simulink model "InverterStartupControl"  (R2022b)
settings: Solver=FixedStepAuto  StartTime=0.0  StopTime=inf  FixedStep=0.005  RelTol=1e-3  EnableMultiTasking=on
undefined symbols (not defined in the file or in its folder): canChannel
libraries: canmsglib x6, canlib x3, simulink x1, motor_interface_lib x1, realtime_pacer_lib x1
settings Model: ExtModeTrigDuration=10  Creator=LinF  LastModifiedBy=LinF
settings SolverCC: AutoInsertRateTranBlk=on
settings OptimizationCC: EnhancedBackFolding=on  PassReuseOutputArgsAs=Individual arguments  ZeroExternalMemoryAtStartup=off  ZeroInternalMemoryAtStartup=off  MaxStackSize=64  OptimizeBlockOrder=speed  DifferentSizesBufferReuse=on  OptimizationCustomize=off  EfficientTunableParamExpr=on
settings DebuggingCC: ParameterTunabilityLossMsg=error
settings HardwareCC: ProdBitPerPointer=32  ProdBitPerSizeT=32  ProdBitPerPtrDiffT=32  ProdLargestAtomicInteger=Long  ProdLargestAtomicFloat=Double  ProdWordSize=32  ProdLongLongMode=on  ProdHWDeviceType=ARM Compatible->ARM Cortex  UseEmbeddedCoderFeatures=off
settings SFSimCC: MATLABDynamicMemAlloc=off
settings RTWCC: Description=Embedded Coder  SystemTargetFile=ert.tlc  HardwareBoard=STM32 Nucleo F767ZI  TLCOptions=-aInlineSetEventsForThisBaseRateFcn=TLC_FALSE -aSuppressMultiTaskScheduler=TLC_FALSE -aRateBasedStepFcn=1  TemplateMakefile=ert_default_tmf  Toolchain=GNU Tools for ARM Embedded Processors
settings CodeAppCC: ForceParamTrailComments=on  IgnoreCustomStorageClasses=off  OperatorAnnotations=on  SimulinkDataObjDesc=on  SFDataObjDesc=on  InsertBlockDesc=on
settings ERTTargetCC: SupportNonInlinedSFcns=on  ExtModeTransport=3  ExtModeStaticAlloc=on  ExtModeStaticAllocSize=2000  ExtModeMexFile=ext_xcp  ExtModeIntrfLevel=Level2 - Open

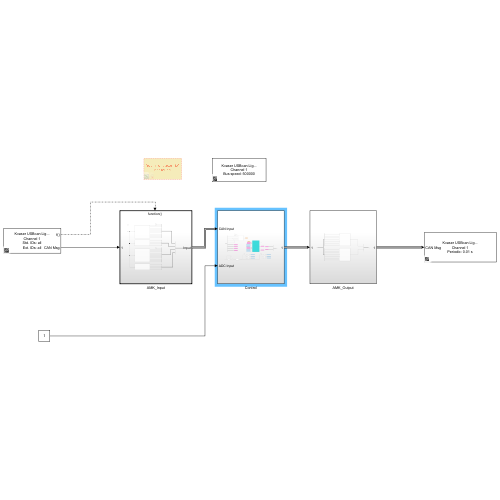
[thumbnail: Simulink's stored preview of the top-level diagram]
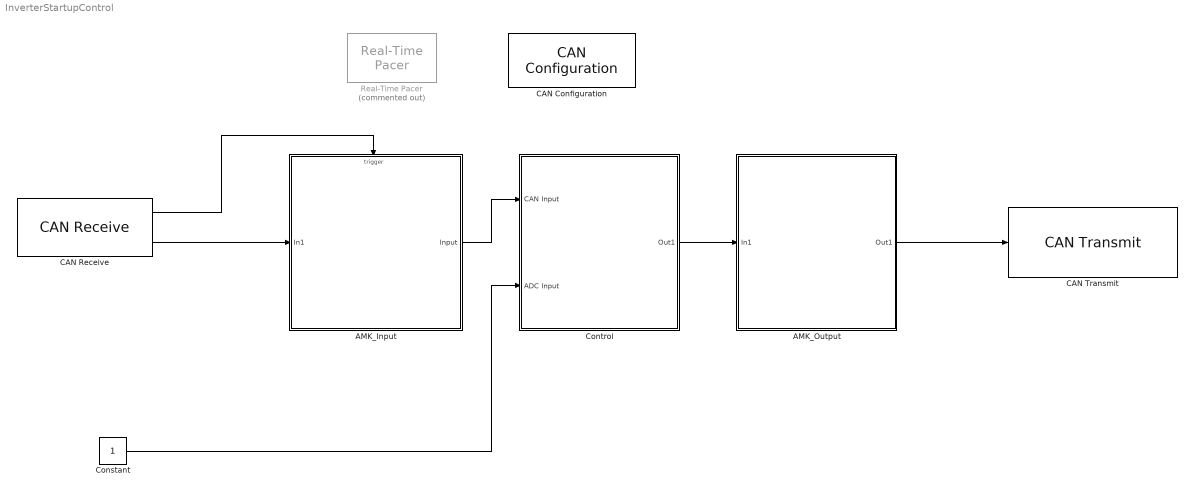
== system InverterStartupControl ==
  AMK_Input : Subsystem  TreatAsAtomicUnit=on
  AMK_Output : Subsystem
  CAN Configuration : canlib/CAN Configuration  BlockHandle=168.0002  Device=Kvaser USBcan Light 1 (Channel 1)  DeviceMenu=Kvaser USBcan Light 1 (Channel 1)  ObjConstructor=canChannel('Kvaser', 'USBcan Light 1', 1)  BusSpeed=500000  EnableBitParameters=off  SJW=4  TSEG1=11  TSEG2=4  NSamples=3  AckMode=Normal
  CAN Receive : canlib/CAN Receive  BlockHandle=169.0002  Device=Kvaser USBcan Light 1 (Channel 1)  DeviceMenu=Kvaser USBcan Light 1 (Channel 1)  ObjConstructor=canChannel('Kvaser', 'USBcan Light 1', 1)  EnableStandardIDsFilter=off  StdIDsCombo=Allow all  StandardIDs=0  EnableExtendedIDsFilter=off  ExtIDsCombo=Allow all  ExtendedIDs=0  SampleTime=0.005  MsgsPerTimestep=all  InternalFilterUpdateStatus=on  BusOutput=off
  CAN Transmit : canlib/CAN Transmit  BlockHandle=172.0002  Device=Kvaser USBcan Light 1 (Channel 1)  DeviceMenu=Kvaser USBcan Light 1 (Channel 1)  ObjConstructor=canChannel('Kvaser', 'USBcan Light 1', 1)  EnableEventTransmit=off  EnablePeriodicTransmit=on  MessagePeriod=0.01
  Constant : Constant
  Control : Subsystem
  Real-Time Pacer : realtime_pacer_lib/Real-Time Pacer  Commented=on  simTimePerRealTime=1
  wires:
  Control/1(Out1) -> AMK_Output/1(In1)
  AMK_Input/1(Input) -> Control/1(CAN Input)
  AMK_Output/1(Out1) -> CAN Transmit/1
  CAN Receive/2 -> AMK_Input/1(In1)
  CAN Receive/1 -> AMK_Input/Trigger
  Constant/1 -> Control/2(ADC Input)

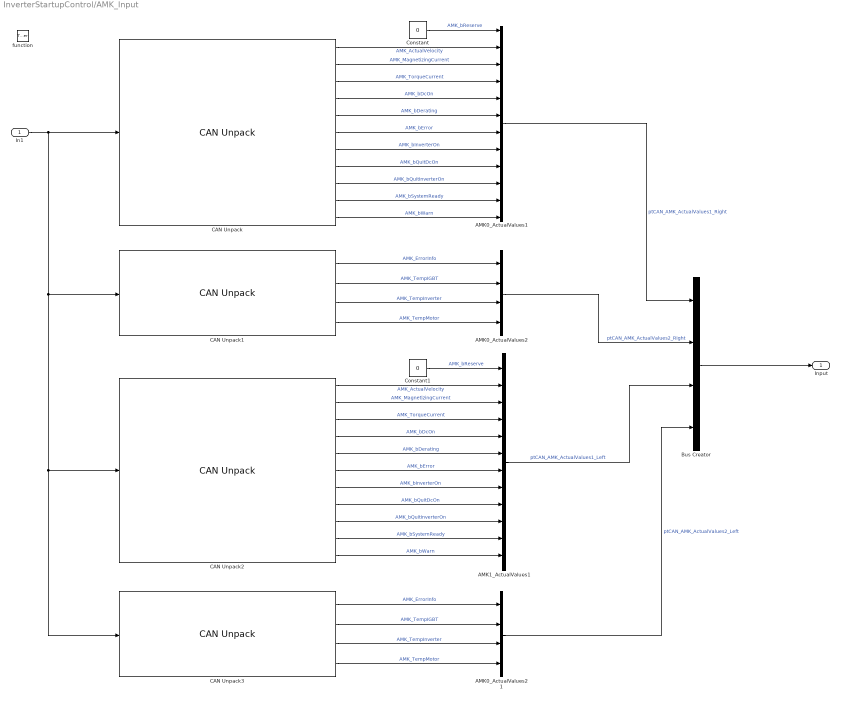
== system InverterStartupControl/AMK_Input ==
  In1 : Inport
  function : TriggerPort  TriggerType=function-call  VariantControl=(inherit)
  "AMK0_ActualValues1 " : BusCreator  Inputs=12
  "AMK0_ActualValues2 " : BusCreator  Inputs=4
  AMK0_ActualValues2 1 : BusCreator  Inputs=4
  AMK1_ActualValues1 : BusCreator  Inputs=12
  Bus Creator : BusCreator  Inputs=4
  CAN Unpack : canmsglib/CAN Unpack  CANdbFile=C:\Users\LinF\Documents\MACFE\Embedded\CAN_Stuff\CAN_Databases\CAN_AMKInverter.dbc  MsgList=AMK0_ActualValues1  MsgName=AMK0_ActualValues1  MsgIDType=Standard (11-bit identifier)  MsgIdentifier=644  MsgLength=8  SignalInfo={'AMK_ActualVelocity','16','16','LE','signed','Standard','0','1','0','-Inf','Inf';'AMK_MagnetizingCurrent','48','16','LE','signed','Standard','0','1','0','-Inf','Inf';'AMK_TorqueCurrent','32','16','LE','signed','Standard','0','1','0','-Inf','Inf';'AMK_bDcOn','12','1','LE','unsigned','Standard','0','1','0','-Inf','Inf';'AMK_bDerating','15','1','LE','unsigned','Standard','0','1','0','-Inf','Inf';'AMK_bError','9','1','LE','unsigned','Standard','0','1','0','-Inf','Inf';'AMK_bInverterOn','14','1','LE','unsigned','Standard','0','1','0','-Inf','Inf';'AMK_bQuitDcOn','11','1','LE','unsigned','Standard','0','1','0','-Inf','Inf';'AMK_bQuitInverterOn','13','1','LE','unsigned','Standard','0','1','0','-Inf','Inf';'AMK_bSystemReady','8','1','LE','unsigned','Standard','0','1','0','-Inf','Inf';'AMK_bWarn','10','1','LE','unsigned','Standard','0','1','0','-Inf','Inf'}  IDPort=off  TimestampPort=off  ErrorPort=off  RemotePort=off  LengthPort=off  StatusPort=off  ApplyMinMax=off
      settings: LibrarySourceBlock=canlib/CAN Unpack  DataFormat=CANdb specified signals
  CAN Unpack1 : canmsglib/CAN Unpack  CANdbFile=C:\Users\LinF\Documents\MACFE\Embedded\CAN_Stuff\CAN_Databases\CAN_AMKInverter.dbc  MsgList=AMK0_ActualValues2  MsgName=AMK0_ActualValues2  MsgIDType=Standard (11-bit identifier)  MsgIdentifier=646  MsgLength=8  SignalInfo={'AMK_ErrorInfo','32','16','LE','unsigned','Standard','0','1','0','0','65535';'AMK_TempIGBT','48','16','LE','signed','Standard','0','0.1','0','-3276.8','3276.7';'AMK_TempInverter','16','16','LE','signed','Standard','0','0.1','0','-3276.8','3276.7';'AMK_TempMotor','0','16','LE','signed','Standard','0','0.1','0','-3276.8','3276.7'}  IDPort=off  TimestampPort=off  ErrorPort=off  RemotePort=off  LengthPort=off  StatusPort=off  ApplyMinMax=off
      settings: LibrarySourceBlock=canlib/CAN Unpack  DataFormat=CANdb specified signals
  CAN Unpack2 : canmsglib/CAN Unpack  CANdbFile=C:\Users\LinF\Documents\MACFE\Embedded\CAN_Stuff\CAN_Databases\CAN_AMKInverter.dbc  MsgList=AMK1_ActualValues1  MsgName=AMK1_ActualValues1  MsgIDType=Standard (11-bit identifier)  MsgIdentifier=645  MsgLength=8  SignalInfo={'AMK_ActualVelocity','16','16','LE','signed','Standard','0','1','0','-Inf','Inf';'AMK_MagnetizingCurrent','48','16','LE','signed','Standard','0','1','0','-Inf','Inf';'AMK_TorqueCurrent','32','16','LE','signed','Standard','0','1','0','-Inf','Inf';'AMK_bDcOn','12','1','LE','unsigned','Standard','0','1','0','-Inf','Inf';'AMK_bDerating','15','1','LE','unsigned','Standard','0','1','0','-Inf','Inf';'AMK_bError','9','1','LE','unsigned','Standard','0','1','0','-Inf','Inf';'AMK_bInverterOn','14','1','LE','unsigned','Standard','0','1','0','-Inf','Inf';'AMK_bQuitDcOn','11','1','LE','unsigned','Standard','0','1','0','-Inf','Inf';'AMK_bQuitInverterOn','13','1','LE','unsigned','Standard','0','1','0','-Inf','Inf';'AMK_bSystemReady','8','1','LE','unsigned','Standard','0','1','0','-Inf','Inf';'AMK_bWarn','10','1','LE','unsigned','Standard','0','1','0','-Inf','Inf'}  IDPort=off  TimestampPort=off  ErrorPort=off  RemotePort=off  LengthPort=off  StatusPort=off  ApplyMinMax=off
      settings: LibrarySourceBlock=canlib/CAN Unpack  DataFormat=CANdb specified signals
  CAN Unpack3 : canmsglib/CAN Unpack  CANdbFile=C:\Users\LinF\Documents\MACFE\Embedded\CAN_Stuff\CAN_Databases\CAN_AMKInverter.dbc  MsgList=AMK1_ActualValues2  MsgName=AMK1_ActualValues2  MsgIDType=Standard (11-bit identifier)  MsgIdentifier=647  MsgLength=8  SignalInfo={'AMK_ErrorInfo','32','16','LE','unsigned','Standard','0','1','0','0','65535';'AMK_TempIGBT','48','16','LE','signed','Standard','0','0.1','0','-3276.8','3276.7';'AMK_TempInverter','16','16','LE','signed','Standard','0','0.1','0','-3276.8','3276.7';'AMK_TempMotor','0','16','LE','signed','Standard','0','0.1','0','-3276.8','3276.7'}  IDPort=off  TimestampPort=off  ErrorPort=off  RemotePort=off  LengthPort=off  StatusPort=off  ApplyMinMax=off
      settings: LibrarySourceBlock=canlib/CAN Unpack  DataFormat=CANdb specified signals
  Constant : Constant  Value=0
  Constant1 : Constant  Value=0
  Input : Outport
  wires:
  In1/1 -> CAN Unpack3/1, CAN Unpack2/1, CAN Unpack1/1, CAN Unpack/1
  CAN Unpack/1 -> "AMK0_ActualValues1 "/2  "AMK_ActualVelocity"
  CAN Unpack/2 -> "AMK0_ActualValues1 "/3  "AMK_MagnetizingCurrent"
  CAN Unpack/3 -> "AMK0_ActualValues1 "/4  "AMK_TorqueCurrent"
  CAN Unpack/4 -> "AMK0_ActualValues1 "/5  "AMK_bDcOn"
  CAN Unpack/5 -> "AMK0_ActualValues1 "/6  "AMK_bDerating"
  CAN Unpack/6 -> "AMK0_ActualValues1 "/7  "AMK_bError"
  CAN Unpack/7 -> "AMK0_ActualValues1 "/8  "AMK_bInverterOn"
  CAN Unpack/8 -> "AMK0_ActualValues1 "/9  "AMK_bQuitDcOn"
  CAN Unpack/9 -> "AMK0_ActualValues1 "/10  "AMK_bQuitInverterOn"
  CAN Unpack/10 -> "AMK0_ActualValues1 "/11  "AMK_bSystemReady"
  CAN Unpack/11 -> "AMK0_ActualValues1 "/12  "AMK_bWarn"
  "AMK0_ActualValues1 "/1 -> Bus Creator/1  "ptCAN_AMK_ActualValues1_Right"
  Bus Creator/1 -> Input/1
  CAN Unpack2/1 -> AMK1_ActualValues1/2  "AMK_ActualVelocity"
  CAN Unpack2/10 -> AMK1_ActualValues1/11  "AMK_bSystemReady"
  CAN Unpack2/6 -> AMK1_ActualValues1/7  "AMK_bError"
  CAN Unpack2/9 -> AMK1_ActualValues1/10  "AMK_bQuitInverterOn"
  CAN Unpack2/2 -> AMK1_ActualValues1/3  "AMK_MagnetizingCurrent"
  CAN Unpack2/3 -> AMK1_ActualValues1/4  "AMK_TorqueCurrent"
  AMK1_ActualValues1/1 -> Bus Creator/3  "ptCAN_AMK_ActualValues1_Left"
  CAN Unpack2/8 -> AMK1_ActualValues1/9  "AMK_bQuitDcOn"
  CAN Unpack2/4 -> AMK1_ActualValues1/5  "AMK_bDcOn"
  CAN Unpack2/5 -> AMK1_ActualValues1/6  "AMK_bDerating"
  CAN Unpack2/11 -> AMK1_ActualValues1/12  "AMK_bWarn"
  CAN Unpack2/7 -> AMK1_ActualValues1/8  "AMK_bInverterOn"
  CAN Unpack1/1 -> "AMK0_ActualValues2 "/1  "AMK_ErrorInfo"
  CAN Unpack1/2 -> "AMK0_ActualValues2 "/2  "AMK_TempIGBT"
  CAN Unpack1/3 -> "AMK0_ActualValues2 "/3  "AMK_TempInverter"
  CAN Unpack1/4 -> "AMK0_ActualValues2 "/4  "AMK_TempMotor"
  "AMK0_ActualValues2 "/1 -> Bus Creator/2  "ptCAN_AMK_ActualValues2_Right"
  CAN Unpack3/1 -> AMK0_ActualValues2 1/1  "AMK_ErrorInfo"
  CAN Unpack3/4 -> AMK0_ActualValues2 1/4  "AMK_TempMotor"
  AMK0_ActualValues2 1/1 -> Bus Creator/4  "ptCAN_AMK_ActualValues2_Left"
  CAN Unpack3/3 -> AMK0_ActualValues2 1/3  "AMK_TempInverter"
  CAN Unpack3/2 -> AMK0_ActualValues2 1/2  "AMK_TempIGBT"
  Constant/1 -> "AMK0_ActualValues1 "/1  "AMK_bReserve"
  Constant1/1 -> AMK1_ActualValues1/1  "AMK_bReserve"

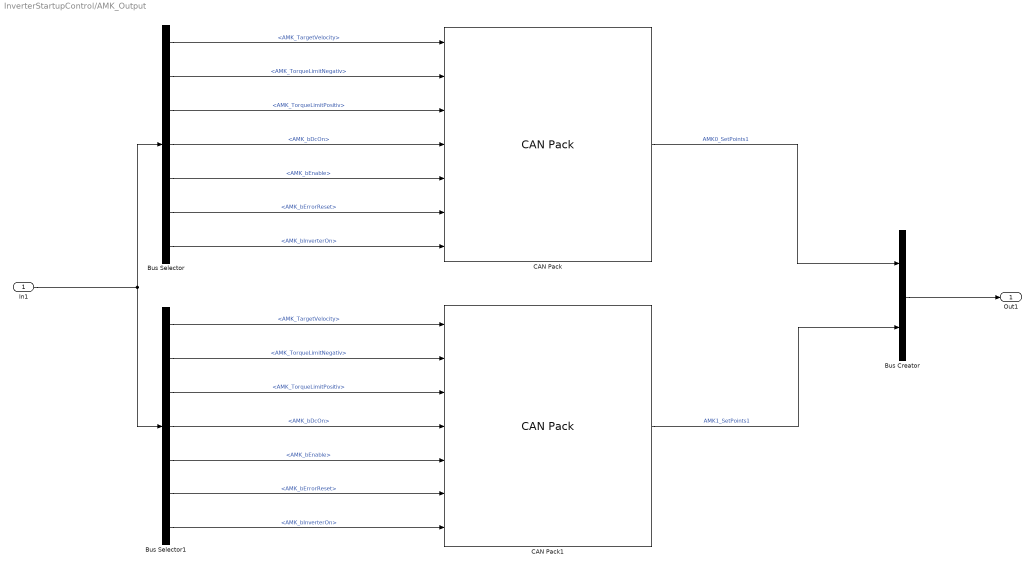
== system InverterStartupControl/AMK_Output ==
  In1 : Inport
  Bus Creator : BusCreator  Inputs=2
  Bus Selector : BusSelector  OutputSignals=ptCAN_AMK_Setpoints1_Right.AMK_TargetVelocity,ptCAN_AMK_Setpoints1_Right.AMK_TorqueLimitNegativ,ptCAN_AMK_Setpoints1_Right.AMK_TorqueLimitPositiv,ptCAN_AMK_Setpoints1_Right.AMK_bDcOn,ptCAN_AMK_Setpoints1_Right.AMK_bEnable,ptCAN_AMK_Setpoints1_Right.AMK_bErrorReset,ptCAN_AMK_Setpoints1_Right.AMK_bInverterOn
  Bus Selector1 : BusSelector  OutputSignals=ptCAN_AMK_Setpoints1_Left.AMK_TargetVelocity,ptCAN_AMK_Setpoints1_Left.AMK_TorqueLimitNegativ,ptCAN_AMK_Setpoints1_Left.AMK_TorqueLimitPositiv,ptCAN_AMK_Setpoints1_Left.AMK_bDcOn,ptCAN_AMK_Setpoints1_Left.AMK_bEnable,ptCAN_AMK_Setpoints1_Left.AMK_bErrorReset,ptCAN_AMK_Setpoints1_Left.AMK_bInverterOn
  CAN Pack : canmsglib/CAN Pack  CANdbFile=C:\Users\LinF\Documents\MACFE\Embedded\CAN_Stuff\CAN_Databases\CAN_AMKInverter.dbc  MsgList=AMK0_SetPoints1  MsgName=AMK0_SetPoints1  MsgIDType=Standard (11-bit identifier)  MsgIdentifier=389  MsgLength=8  Remote=off  ApplyMinMax=off  BusOutput=off  SignalInfo={'AMK_TargetVelocity','16','16','LE','signed','Standard','0','1','0','-Inf','Inf';'AMK_TorqueLimitNegativ','48','16','LE','signed','Standard','0','1','0','-Inf','Inf';'AMK_TorqueLimitPositiv','32','16','LE','signed','Standard','0','1','0','-Inf','Inf';'AMK_bDcOn','9','1','LE','unsigned','Standard','0','1','0','-Inf','Inf';'AMK_bEnable','10','1','LE','unsigned','Standard','0','1','0','-Inf','Inf';'AMK_bErrorReset','11','1','LE','unsigned','Standard','0','1','0','-Inf','Inf';'AMK_bInverterOn','8','1','LE','unsigned','Standard','0','1','0','-Inf','Inf'}
      settings: LibrarySourceBlock=canlib/CAN Pack  DataFormat=CANdb specified signals
  CAN Pack1 : canmsglib/CAN Pack  CANdbFile=C:\Users\LinF\Documents\MACFE\Embedded\CAN_Stuff\CAN_Databases\CAN_AMKInverter.dbc  MsgList=AMK1_SetPoints1  MsgName=AMK1_SetPoints1  MsgIDType=Standard (11-bit identifier)  MsgIdentifier=390  MsgLength=8  Remote=off  ApplyMinMax=off  BusOutput=off  SignalInfo={'AMK_TargetVelocity','16','16','LE','signed','Standard','0','1','0','-Inf','Inf';'AMK_TorqueLimitNegativ','48','16','LE','signed','Standard','0','1','0','-Inf','Inf';'AMK_TorqueLimitPositiv','32','16','LE','signed','Standard','0','1','0','-Inf','Inf';'AMK_bDcOn','9','1','LE','unsigned','Standard','0','1','0','-Inf','Inf';'AMK_bEnable','10','1','LE','unsigned','Standard','0','1','0','-Inf','Inf';'AMK_bErrorReset','11','1','LE','unsigned','Standard','0','1','0','-Inf','Inf';'AMK_bInverterOn','8','1','LE','unsigned','Standard','0','1','0','-Inf','Inf'}
      settings: LibrarySourceBlock=canlib/CAN Pack  DataFormat=CANdb specified signals
  Out1 : Outport
  wires:
  In1/1 -> Bus Selector/1, Bus Selector1/1
  CAN Pack/1 -> Bus Creator/1  "AMK0_SetPoints1"
  CAN Pack1/1 -> Bus Creator/2  "AMK1_SetPoints1"
  Bus Selector/7 -> CAN Pack/7  "<AMK_bInverterOn>"
  Bus Selector/4 -> CAN Pack/4  "<AMK_bDcOn>"
  Bus Selector/5 -> CAN Pack/5  "<AMK_bEnable>"
  Bus Selector/6 -> CAN Pack/6  "<AMK_bErrorReset>"
  Bus Selector/1 -> CAN Pack/1  "<AMK_TargetVelocity>"
  Bus Selector/3 -> CAN Pack/3  "<AMK_TorqueLimitPositiv>"
  Bus Selector/2 -> CAN Pack/2  "<AMK_TorqueLimitNegativ>"
  Bus Creator/1 -> Out1/1
  Bus Selector1/1 -> CAN Pack1/1  "<AMK_TargetVelocity>"
  Bus Selector1/3 -> CAN Pack1/3  "<AMK_TorqueLimitPositiv>"
  Bus Selector1/2 -> CAN Pack1/2  "<AMK_TorqueLimitNegativ>"
  Bus Selector1/4 -> CAN Pack1/4  "<AMK_bDcOn>"
  Bus Selector1/5 -> CAN Pack1/5  "<AMK_bEnable>"
  Bus Selector1/6 -> CAN Pack1/6  "<AMK_bErrorReset>"
  Bus Selector1/7 -> CAN Pack1/7  "<AMK_bInverterOn>"

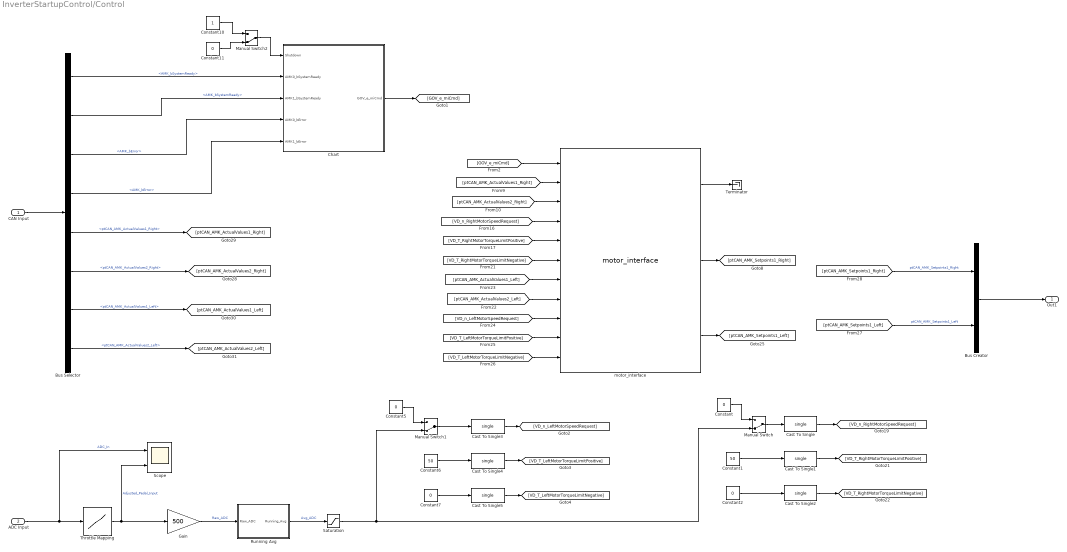
== system InverterStartupControl/Control ==
  CAN Input : Inport
  ADC Input : Inport  Port=2
  Bus Creator : BusCreator  Inputs=2
  Bus Selector : BusSelector  OutputSignals=ptCAN_AMK_ActualValues1_Right.AMK_bSystemReady,ptCAN_AMK_ActualValues1_Left.AMK_bSystemReady,ptCAN_AMK_ActualValues1_Right.AMK_bError,ptCAN_AMK_ActualValues1_Left.AMK_bError,ptCAN_AMK_ActualValues1_Right,ptCAN_AMK_ActualValues2_Right,ptCAN_AMK_ActualValues1_Left,ptCAN_AMK_ActualValues2_Left
  Cast To Single{,1..5} (6 alike) : DataTypeConversion  OutDataTypeStr=single  SaturateOnIntegerOverflow=off  RndMeth=Floor
  Chart : Stateflow chart  TreatAsAtomicUnit=on
  Constant{,2,5,7,11} (5 alike) : Constant  Value=0
  Constant1 : Constant  Value=50
  Constant10 : Constant
  Constant6 : Constant  Value=50
  Gain : Gain  Gain=500
  Manual Switch : ManualSwitch  CurrentSetting=0
  Manual Switch1 : ManualSwitch  CurrentSetting=0
  Manual Switch2 : ManualSwitch  CurrentSetting=0
  Running Avg : Subsystem
  Saturation : Saturate  UpperLimit=500  LowerLimit=0
  Scope : Scope  NumInputPorts=2
  Terminator : Terminator
  Throttle Mapping : Lookup_n-D  NumberOfTableDimensions=1  BreakpointsForDimension1=[0:0.025:1]  Table=[0 0 0 linspace(0,1,36) 1 1]  TableMax=[1]  InternalRulePriority=Speed  RndMeth=Simplest
  motor_interface : motor_interface_lib/motor_interface  SystemSampleTime=-1  VariantActivationTime=update diagram  Latency=0  AutoFrameSizeCalculation=off
  Out1 : Outport
  wires:
  [VD_T_RightMotorTorqueLimitPositive] -> motor_interface/5
  [ptCAN_AMK_ActualValues2_Right] -> motor_interface/3
  [ptCAN_AMK_ActualValues2_Left] -> motor_interface/8
  [VD_n_LeftMotorSpeedRequest] -> motor_interface/9
  [VD_T_LeftMotorTorqueLimitNegative] -> motor_interface/11
  [VD_T_RightMotorTorqueLimitNegative] -> motor_interface/6
  motor_interface/2 -> [ptCAN_AMK_Setpoints1_Right]
  motor_interface/3 -> [ptCAN_AMK_Setpoints1_Left]
  [VD_T_LeftMotorTorqueLimitPositive] -> motor_interface/10
  [VD_n_RightMotorSpeedRequest] -> motor_interface/4
  [ptCAN_AMK_ActualValues1_Left] -> motor_interface/7
  motor_interface/1 -> Terminator/1
  [GOV_e_miCmd] -> motor_interface/1
  [ptCAN_AMK_ActualValues1_Right] -> motor_interface/2
  CAN Input/1 -> Bus Selector/1
  Bus Selector/6 -> [ptCAN_AMK_ActualValues2_Right]  "<ptCAN_AMK_ActualValues2_Right>"
  Constant2/1 -> Cast To Single2/1
  Bus Selector/8 -> [ptCAN_AMK_ActualValues2_Left]  "<ptCAN_AMK_ActualValues2_Left>"
  Constant7/1 -> Cast To Single5/1
  Manual Switch1/1 -> Cast To Single3/1
  Chart/1(GOV_e_miCmd) -> [GOV_e_miCmd]
  [ptCAN_AMK_Setpoints1_Right] -> Bus Creator/1  "ptCAN_AMK_Setpoints1_Right"
  [ptCAN_AMK_Setpoints1_Left] -> Bus Creator/2  "ptCAN_AMK_Setpoints1_Left"
  Bus Creator/1 -> Out1/1
  Bus Selector/5 -> [ptCAN_AMK_ActualValues1_Right]  "<ptCAN_AMK_ActualValues1_Right>"
  Bus Selector/1 -> Chart/2(AMK0_bSystemReady)  "<AMK_bSystemReady>"
  Bus Selector/3 -> Chart/4(AMK0_bError)  "<AMK_bError>"
  Constant/1 -> Manual Switch/1
  Manual Switch/1 -> Cast To Single/1
  Constant10/1 -> Manual Switch2/1
  Constant11/1 -> Manual Switch2/2
  Manual Switch2/1 -> Chart/1(Shutdown)
  Bus Selector/7 -> [ptCAN_AMK_ActualValues1_Left]  "<ptCAN_AMK_ActualValues1_Left>"
  Cast To Single/1 -> [VD_n_RightMotorSpeedRequest]
  Cast To Single1/1 -> [VD_T_RightMotorTorqueLimitPositive]
  Cast To Single2/1 -> [VD_T_RightMotorTorqueLimitNegative]
  Cast To Single3/1 -> [VD_n_LeftMotorSpeedRequest]
  Cast To Single4/1 -> [VD_T_LeftMotorTorqueLimitPositive]
  Cast To Single5/1 -> [VD_T_LeftMotorTorqueLimitNegative]
  Bus Selector/2 -> Chart/3(AMK1_bSystemReady)  "<AMK_bSystemReady>"
  Bus Selector/4 -> Chart/5(AMK1_bError)  "<AMK_bError>"
  Constant5/1 -> Manual Switch1/1
  Throttle Mapping/1 -> Scope/2, Gain/1  "Adjusted_Pedal_Input"
  Gain/1 -> Running Avg/1(Raw_ADC)  "Raw_ADC"
  Saturation/1 -> Manual Switch/2, Manual Switch1/2
  ADC Input/1 -> Scope/1, Throttle Mapping/1  "ADC_In"
  Running Avg/1(Running_Avg) -> Saturation/1  "Avg_ADC"
  Constant1/1 -> Cast To Single1/1
  Constant6/1 -> Cast To Single4/1

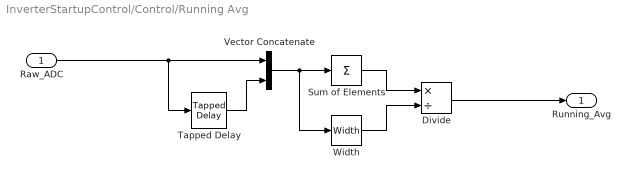
== system InverterStartupControl/Control/Running Avg ==
  Raw_ADC : Inport
  Divide : Product  Inputs=*/
  Sum of Elements : Sum  Inputs=+
  Tapped Delay : simulink/Discrete/Tapped Delay  vinit=0  samptime=-1  NumDelays=5  DelayOrder=Oldest  includeCurrent=off
  Vector Concatenate : Concatenate
  Width : Width
  Running_Avg : Outport
  wires:
  Divide/1 -> Running_Avg/1
  Vector Concatenate/1 -> Width/1, Sum of Elements/1
  Raw_ADC/1 -> Vector Concatenate/1, Tapped Delay/1
  Width/1 -> Divide/2
  Tapped Delay/1 -> Vector Concatenate/2
  Sum of Elements/1 -> Divide/1

== stateflow chart InverterStartupControl/Control/Chart ==
  state Init
    en:
    GOV_e_miCmd = MI_CMD.CMD_INIT;
  state Run
    en:
    GOV_e_miCmd = MI_CMD.CMD_STARTUP;
  state Error0
    en:
    GOV_e_miCmd = MI_CMD.ERR_RESET;
  state Error1
    en:
    GOV_e_miCmd = MI_CMD.ERR_RESET;
  state Shutdown
    en:
    GOV_e_miCmd = MI_CMD.CMD_SHUTDOWN;
  (default) -> Init
  Shutdown -> Init : [Shutdown == 0]
  Init -> Run : [(AMK0_bSystemReady == 1 && AMK1_bSystemReady == 1) && Shutdown == 0]
  Run -> Error0 [order 1] : [AMK0_bError == 1]
  Error0 -> Run : [AMK0_bError == 0]
  Run -> Error1 [order 3] : [AMK1_bError == 1]
  Error1 -> Run : [AMK1_bError == 0]
  Run -> Shutdown [order 2] : [Shutdown == 1]
  data: Shutdown input; GOV_e_miCmd output; AMK0_bSystemReady input; AMK1_bSystemReady input; AMK0_bError input; AMK1_bError input
